simulink model "MPC_circle_tracking"  (R2023a)
settings: Solver=VariableStepAuto  StartTime=0.0  StopTime=40  FixedStep=0.001  RelTol=1e-3
libraries: slpidlib x2, Solver_SF x1
settings Model: Creator=ASUS  LastModifiedBy=69546
settings SolverCC: AlgebraicLoopSolver=TrustRegion
settings DebuggingCC: UnconnectedInputMsg=warning  UnconnectedOutputMsg=warning  UnconnectedLineMsg=warning
settings ModelReferenceCC: EnableRefExpFcnMdlSchedulingChecks=on
settings SFSimCC: CustomCodeUndefinedFunction=UseInterfaceOnly

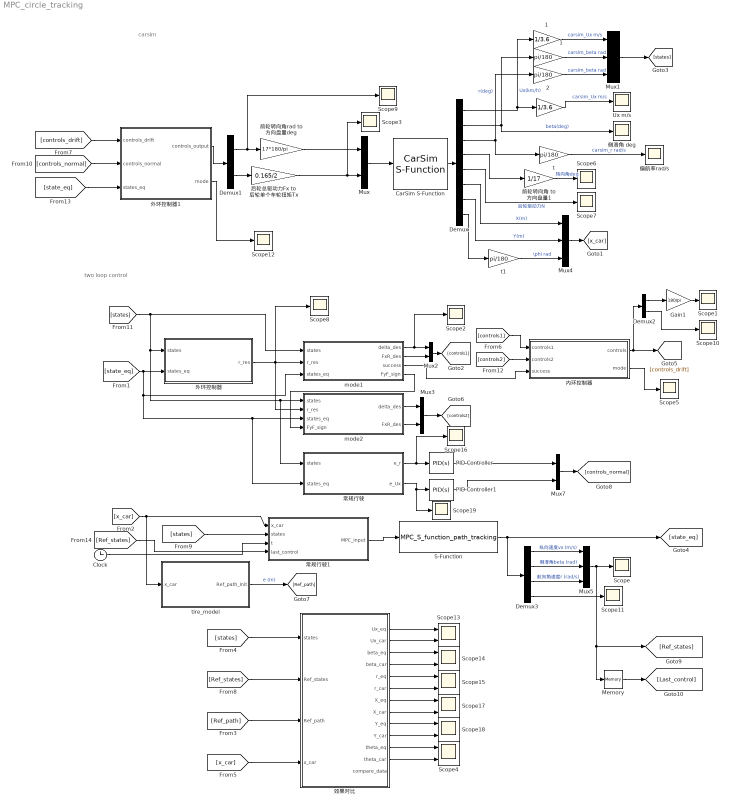
== system MPC_circle_tracking ==
  note: carsim
  note: two loop control
  " " : Gain  Gain=1/3.6
  " 1" : Gain  Gain=1/3.6
  " 1" : Gain  Gain=pi/180
  " 2" : Gain  Gain=pi/180
  " t" : Gain  Gain=pi/180
  " t1" : Gain  Gain=pi/180
  CarSim S-Function : Solver_SF/CarSim S-Function  Priority=1  SIMFILE=simfile.sim  Run_RTs=off  vs_state_ind=Run  StopMode_ind=Vehicle Model
  Clock : Clock
  Demux : Demux  Outputs=8
  Demux1 : Demux  Outputs=[1 1]
  Demux2 : Demux  Outputs=2
  Demux3 : Demux
  Gain1 : Gain  Gain=180/pi
  Memory : Memory
  Mux{,2..3,7} (4 alike) : Mux  Inputs=2
  Mux1 : Mux  Inputs=3
  Mux4 : Mux  Inputs=3
  Mux5 : Mux  Inputs=3
  PID Controller : slpidlib/PID Controller  Controller=PID  Form=Parallel  TimeDomain=Continuous-time  UseExternalTs=off  SampleTime=-1  IntegratorMethod=Forward Euler  FilterMethod=Forward Euler  ControllerParametersSource=internal  P=3  I=1  UseKiTs=off  D=0  N=100  UseFilter=on  TunerSelectOption=Transfer Function Based (PID Tuner App)  InitialConditionSource=internal  InitialConditionForIntegrator=0  InitialConditionForFilter=0  DifferentiatorICPrevScaledInput=0  ExternalReset=none  TrackingMode=off  Kt=1  LimitOutput=on  SatLimitsSource=internal  UpperSaturationLimit=30*pi/180  LowerSaturationLimit=-30*pi/180  LinearizeAsGain=off  AntiWindupMode=none  Kb=1  LimitIntegrator=off  UpperIntegratorSaturationLimit=inf  LowerIntegratorSaturationLimit=-inf  POutMin=[]  POutMax=[]  IOutMin=[]  IOutMax=[]  DOutMin=[]  DOutMax=[]  NOutMin=[]  NOutMax=[]  SumOutMin=[]  SumOutMax=[]  SaturationOutMin=[]  SaturationOutMax=[]  PParamMin=[]  PParamMax=[]  IParamMin=[]  IParamMax=[]  DParamMin=[]  DParamMax=[]  NParamMin=[]  NParamMax=[]  KbParamMin=[]  KbParamMax=[]  KtParamMin=[]  KtParamMax=[]  KbOutMin=[]  KbOutMax=[]  KtOutMin=[]  KtOutMax=[]  IntegratorOutMin=[]  IntegratorOutMax=[]  FilterOutMin=[]  FilterOutMax=[]  SumI1OutMin=[]  SumI1OutMax=[]  SumI2OutMin=[]  SumI2OutMax=[]  SumI3OutMin=[]  SumI3OutMax=[]  SumI4OutMin=[]  SumI4OutMax=[]  SumDOutMin=[]  SumDOutMax=[]  DifferentiatorOutMin=[]  DifferentiatorOutMax=[]  FilterDiffOutCoefMin=[]  FilterDiffOutCoefMax=[]  ReciprocalOutMin=[]  ReciprocalOutMax=[]  SumDenOutMin=[]  SumDenOutMax=[]  SumNumOutMin=[]  SumNumOutMax=[]  DivideOutMin=[]  DivideOutMax=[]  UdiffTsProdOutMin=[]  UdiffTsProdOutMax=[]  NTsProdOutMin=[]  NTsProdOutMax=[]  UintegralTsProdOutMin=[]  UintegralTsProdOutMax=[]  UngainTsProdOutMin=[]  UngainTsProdOutMax=[]  ClampingZeroOutDataTypeStr=Inherit: Inherit via back propagation  ClampingZeroOutMin=[]  ClampingZeroOutMax=[]  FilterDenConstantOutDataTypeStr=Inherit: Inherit via back propagation  FilterDenConstantOutMin=[]  FilterDenConstantOutMax=[]  PCopyOutDataTypeStr=Inherit: Inherit via back propagation  PCopyOutMin=[]  PCopyOutMax=[]  NCopyOutDataTypeStr=Inherit: Inherit via back propagation  NCopyOutMin=[]  NCopyOutMax=[]  IntegratorContinuousStateAttributes=''  IntegratorStateMustResolveToSignalObject=off  IntegratorRTWStateStorageClass=Auto  FilterContinuousStateAttributes=''  FilterStateMustResolveToSignalObject=off  FilterRTWStateStorageClass=Auto  ParallelPVariant=InternalParameters  IdealPVariant=Disabled  IVariant=InternalParameters  DVariant=InternalParameters  IntegratorVariant=Continuous  SatVariant=Enabled  AWVariant=Passthrough  PCopyVariant=Disabled  TRVariant=Disabled  FdbkBlocksVariant=Forward  IdealPFdbkVariant=Disabled  SatFdbkVariant=Disabled  DerivativeFilterVariant=ContFilter  NVariant=InternalParameters  NCopyVariant=Disabled  FilterICVariant=InternalICsFilter  IntegratorICVariant=InternalICs  ExternalResetVariant=Disabled  TRSumVariant=Passthrough  SumFdbkVariant=Disabled  SumVariant=Sum_PID  TsampFilterVariant=InternalTs  TsampNgainVariant=Passthrough  TsampIntegralVariant=Disabled_SignalSpec  ExternalSaturationOutDataTypeStr=Inherit: Same as second input
  PID Controller1 : slpidlib/PID Controller  Controller=PID  Form=Parallel  TimeDomain=Continuous-time  UseExternalTs=off  SampleTime=-1  IntegratorMethod=Forward Euler  FilterMethod=Forward Euler  ControllerParametersSource=internal  P=1000  I=50  UseKiTs=off  D=0  N=100  UseFilter=on  TunerSelectOption=Transfer Function Based (PID Tuner App)  InitialConditionSource=internal  InitialConditionForIntegrator=0  InitialConditionForFilter=0  DifferentiatorICPrevScaledInput=0  ExternalReset=none  TrackingMode=off  Kt=1  LimitOutput=on  SatLimitsSource=internal  UpperSaturationLimit=4000  LowerSaturationLimit=-4000  LinearizeAsGain=on  AntiWindupMode=none  Kb=1  LimitIntegrator=off  UpperIntegratorSaturationLimit=inf  LowerIntegratorSaturationLimit=-inf  POutMin=[]  POutMax=[]  IOutMin=[]  IOutMax=[]  DOutMin=[]  DOutMax=[]  NOutMin=[]  NOutMax=[]  SumOutMin=[]  SumOutMax=[]  SaturationOutMin=[]  SaturationOutMax=[]  PParamMin=[]  PParamMax=[]  IParamMin=[]  IParamMax=[]  DParamMin=[]  DParamMax=[]  NParamMin=[]  NParamMax=[]  KbParamMin=[]  KbParamMax=[]  KtParamMin=[]  KtParamMax=[]  KbOutMin=[]  KbOutMax=[]  KtOutMin=[]  KtOutMax=[]  IntegratorOutMin=[]  IntegratorOutMax=[]  FilterOutMin=[]  FilterOutMax=[]  SumI1OutMin=[]  SumI1OutMax=[]  SumI2OutMin=[]  SumI2OutMax=[]  SumI3OutMin=[]  SumI3OutMax=[]  SumI4OutMin=[]  SumI4OutMax=[]  SumDOutMin=[]  SumDOutMax=[]  DifferentiatorOutMin=[]  DifferentiatorOutMax=[]  FilterDiffOutCoefMin=[]  FilterDiffOutCoefMax=[]  ReciprocalOutMin=[]  ReciprocalOutMax=[]  SumDenOutMin=[]  SumDenOutMax=[]  SumNumOutMin=[]  SumNumOutMax=[]  DivideOutMin=[]  DivideOutMax=[]  UdiffTsProdOutMin=[]  UdiffTsProdOutMax=[]  NTsProdOutMin=[]  NTsProdOutMax=[]  UintegralTsProdOutMin=[]  UintegralTsProdOutMax=[]  UngainTsProdOutMin=[]  UngainTsProdOutMax=[]  ClampingZeroOutDataTypeStr=Inherit: Inherit via back propagation  ClampingZeroOutMin=[]  ClampingZeroOutMax=[]  FilterDenConstantOutDataTypeStr=Inherit: Inherit via back propagation  FilterDenConstantOutMin=[]  FilterDenConstantOutMax=[]  PCopyOutDataTypeStr=Inherit: Inherit via back propagation  PCopyOutMin=[]  PCopyOutMax=[]  NCopyOutDataTypeStr=Inherit: Inherit via back propagation  NCopyOutMin=[]  NCopyOutMax=[]  IntegratorContinuousStateAttributes=''  IntegratorStateMustResolveToSignalObject=off  IntegratorRTWStateStorageClass=Auto  FilterContinuousStateAttributes=''  FilterStateMustResolveToSignalObject=off  FilterRTWStateStorageClass=Auto  ParallelPVariant=InternalParameters  IdealPVariant=Disabled  IVariant=InternalParameters  DVariant=InternalParameters  IntegratorVariant=Continuous  SatVariant=Enabled  AWVariant=Passthrough  PCopyVariant=Disabled  TRVariant=Disabled  FdbkBlocksVariant=Forward  IdealPFdbkVariant=Disabled  SatFdbkVariant=Disabled  DerivativeFilterVariant=ContFilter  NVariant=InternalParameters  NCopyVariant=Disabled  FilterICVariant=InternalICsFilter  IntegratorICVariant=InternalICs  ExternalResetVariant=Disabled  TRSumVariant=Passthrough  SumFdbkVariant=Disabled  SumVariant=Sum_PID  TsampFilterVariant=InternalTs  TsampNgainVariant=Passthrough  TsampIntegralVariant=Disabled_SignalSpec  ExternalSaturationOutDataTypeStr=Inherit: Same as second input
  S-Function : S-Function  FunctionName=MPC_S_function_path_tracking  SFunctionDeploymentMode=off  EnableBusSupport=off
  Scope{,1..3,5..12,16,19} (14 alike) : Scope
  Scope{4,13..15,17..18} (6 alike) : Scope  NumInputPorts=2
  Ux m/s : Scope
  mode1 : MATLAB Function  TreatAsAtomicUnit=on
  mode2 : MATLAB Function  TreatAsAtomicUnit=on
  tire_model : MATLAB Function  TreatAsAtomicUnit=on
  侧滑角 deg : Scope
  偏航率rad/s : Scope
  内环控制器 : MATLAB Function  TreatAsAtomicUnit=on
  前轮转向角 to 方向盘量1 : Gain  Gain=1/17
  前轮转向角rad to 方向盘量deg : Gain  Gain=17*180/pi
  后轮总驱动力Fx to 后轮单个车轮扭矩Tx : Gain  Gain=0.165/2
  外环控制器 : MATLAB Function  TreatAsAtomicUnit=on
  外环控制器1 : MATLAB Function  TreatAsAtomicUnit=on
  常规行驶 : MATLAB Function  TreatAsAtomicUnit=on
  常规行驶1 : MATLAB Function  TreatAsAtomicUnit=on
  效果对比 : MATLAB Function  TreatAsAtomicUnit=on
  wires:
  内环控制器/1(controls) -> [controls_drift], Demux2/1
  mode1/1(delta_des) -> Scope2/1, Mux2/1
  Gain1/1 -> Scope1/1
  Demux2/2 -> Scope10/1
  Mux2/1 -> [controls1]
  Demux2/1 -> Gain1/1
  [controls2] -> 内环控制器/2(controls2)
  [states] -> 常规行驶/1(states), mode2/1(states), 外环控制器/1(states), mode1/1(states)
  mode2/1(delta_des) -> Mux3/1
  mode1/2(FxR_des) -> Mux2/2
  Mux3/1 -> [controls2]
  mode2/2(FxR_des) -> Mux3/2
  内环控制器/2(mode) -> Scope5/1
  mode1/3(success) -> 内环控制器/3(success)
  [controls1] -> 内环控制器/1(controls1)
  外环控制器/1(r_res) -> mode2/2(r_res), mode1/2(r_res), Scope8/1
  " t"/1 -> 偏航率rad/s/1  "carsim_r rad/s"
  " "/1 -> Ux m/s/1  "carsim_Ux m/s"
  " 1"/1 -> Mux1/2  "carsim_beta rad"
  " 2"/1 -> Mux1/3  "carsim_beta rad"
  Demux1/2 -> 后轮总驱动力Fx to 后轮单个车轮扭矩Tx/1
  Demux/1 -> " 1"/1, " "/1  "Ux(km/h)"
  Demux/5 -> Scope7/1  "后轮驱动力N"
  Demux/4 -> 前轮转向角 to 方向盘量1/1
  Mux/1 -> CarSim S-Function/1
  Mux1/1 -> [states]
  CarSim S-Function/1 -> Demux/1
  " 1"/1 -> Mux1/1  "carsim_Ux m/s"
  前轮转向角 to 方向盘量1/1 -> Scope6/1  "转向角deg"
  Demux/3 -> " 2"/1, " t"/1  "r(deg)"
  Demux/2 -> " 1"/1, 侧滑角 deg/1  "beta(deg)"
  Demux1/1 -> Scope9/1, 前轮转向角rad to 方向盘量deg/1
  mode1/4(FyF_sign) -> mode2/4(FyF_sign)
  Demux/8 -> " t1"/1
  " t1"/1 -> Mux4/3  "\\phi rad"
  Mux4/1 -> [x_car]
  [state_eq] -> 常规行驶/2(states_eq), mode2/3(states_eq), mode1/3(states_eq), 外环控制器/2(states_eq)
  S-Function/1 -> Demux3/1, [state_eq]
  Demux/6 -> Mux4/1  "X(m)"
  Demux/7 -> Mux4/2  "Y(m)"
  Demux3/1 -> Mux5/1  "纵向速度vx (m/s)"
  Demux3/2 -> Mux5/2  "侧滑角beta (rad)"
  Demux3/3 -> Mux5/3  "航向角速度r (rad/s)"
  Mux5/1 -> Memory/1, [Ref_states], Scope/1
  常规行驶/1(e_r) -> Scope16/1, PID Controller/1
  常规行驶/2(e_Ux) -> Scope19/1, PID Controller1/1
  Mux7/1 -> [controls_normal]
  常规行驶1/1(MPC_input) -> S-Function/1
  tire_model/1(Ref_path_Init) -> [Ref_path]  "e (m)"
  [x_car] -> tire_model/1(x_car), 常规行驶1/1(x_car)
  效果对比/4(beta_car) -> Scope14/2
  效果对比/6(r_car) -> Scope15/2
  效果对比/8(X_car) -> Scope17/2
  效果对比/7(X_eq) -> Scope17/1
  效果对比/11(theta_eq) -> Scope4/1
  效果对比/12(theta_car) -> Scope4/2
  [x_car] -> 效果对比/4(x_car)
  效果对比/10(Y_car) -> Scope18/2
  效果对比/3(beta_eq) -> Scope14/1
  效果对比/9(Y_eq) -> Scope18/1
  [states] -> 效果对比/1(states)
  效果对比/5(r_eq) -> Scope15/1
  效果对比/2(Ux_car) -> Scope13/2
  [Ref_path] -> 效果对比/3(Ref_path)
  效果对比/1(Ux_eq) -> Scope13/1
  Demux3/4 -> Scope11/1
  PID Controller1/1 -> Mux7/2
  Clock/1 -> 常规行驶1/3(t)
  后轮总驱动力Fx to 后轮单个车轮扭矩Tx/1 -> Scope3/1, Mux/2
  前轮转向角rad to 方向盘量deg/1 -> Mux/1
  [Ref_states] -> 效果对比/2(Ref_states)
  [states] -> 常规行驶1/2(states)
  [controls_drift] -> 外环控制器1/1(controls_drift)
  外环控制器1/1(controls_output) -> Demux1/1
  [controls_normal] -> 外环控制器1/2(controls_normal)
  [state_eq] -> 外环控制器1/3(states_eq)
  外环控制器1/2(mode) -> Scope12/1
  PID Controller/1 -> Mux7/1
  [Ref_states] -> 常规行驶1/4(last_control)
  Memory/1 -> [Last_control]

== matlab function MPC_circle_tracking/效果对比 ==
  data: Ux_eq output; states input; Ref_states input; Ref_path input; x_car input; Ux_car output; beta_eq output; beta_car output; r_eq output; r_car output; X_eq output; X_car output; Y_eq output; Y_car output; theta_eq output; theta_car output; compare_data output
 function [Ux_eq,Ux_car,beta_eq,beta_car,r_eq,r_car,X_eq,X_car,Y_eq,Y_car,theta_eq,theta_car,compare_data] = output_compare(states,Ref_states,Ref_path,x_car)
        %期望值
        
        X_eq=Ref_path(1);
        Y_eq=Ref_path(2);
        theta_eq=Ref_path(3);
        Ux_eq=Ref_path(4);
        beta_eq=atan2(Ref_path(5),Ux_eq);
        r_eq=Ref_path(6);
        % Ux_eq=Ref_states(1);
        % beta_eq=Ref_states(2);
        % r_eq=Ref_states(3);
        V_eq=Ux_eq/( cos(beta_eq)+eps );
        %实际值
        Ux_car=states(1);
        beta_car=states(2);
        r_car=states(3);
        
        X_car=x_car(1);
        Y_car=x_car(2);
        theta_car=x_car(3);

        V_car=Ux_car/( cos(beta_car)+eps );
        compare_data=[Ux_eq,Ux_car,beta_eq,beta_car,r_eq,r_car,X_eq,X_car,Y_eq,Y_car,theta_eq,theta_car] ;
        
end

== matlab function MPC_circle_tracking/外环控制器1 ==
  data: controls_output output; controls_drift input; controls_normal input; states_eq input; mode output
function [controls_output,mode] = outloop_control(controls_drift,controls_normal,states_eq)
        %车辆参数及控制器相关参数都在car_parameters文件中配置
        beta_eq=states_eq(2)   ;
        %常规控制器
        if abs(beta_eq)<0.2
            controls_output=controls_normal;
            mode=0;
         %漂移控制器
        else
            controls_output=controls_drift;
            mode=1;
        end

        
end

== matlab function MPC_circle_tracking/常规行驶 ==
  data: e_r output; states input; e_Ux output; states_eq input

function [e_r,e_Ux] = normal(states,states_eq)


    Ux_eq=states_eq(1)    ;
    beta_eq=states_eq(2)    ;
    r_eq=states_eq(3) ;

    Ux = states(1);
    beta=states(2)    ;
    r = states(3);

    e_Ux = -(Ux-Ux_eq);
    e_r = -(r-r_eq)-1*(beta-beta_eq);


end

== matlab function MPC_circle_tracking/tire_model ==
  data: Ref_path_Init output; x_car input
function Ref_path_Init  = tire_model(x_car)
    Ref_path_Init=[0;0;0;0;0;0] ;
    currentPosition=[x_car(1),x_car(2)];
    nearestPoint = findNearestPoint(currentPosition,x_car(3),0);
    %初始最近跟踪匹配点
    X_r=nearestPoint(1);
    Y_r=nearestPoint(2);
    theta_r=nearestPoint(3);  
    Ux_r=nearestPoint(4);
    Uy_r=nearestPoint(5);
    r_r=nearestPoint(6);  
    %最近跟踪点的参考车辆状态
    Ref_path_Init(1)=X_r;
    Ref_path_Init(2)=Y_r;
    Ref_path_Init(3)=theta_r;  
    Ref_path_Init(4)=Ux_r;
    Ref_path_Init(5)=Uy_r;
    Ref_path_Init(6)=r_r;  

             
end

== matlab function MPC_circle_tracking/内环控制器 ==
  data: controls output; controls1 input; controls2 input; success input; mode output
function [controls, mode] = innerloop_control(controls1,controls2,success)
    % Mode 2 - Drive force mode
    if success
        controls=controls1;
        mode = 1;
    else
        controls=controls2;
        mode = 2;
    end
    
end

== matlab function MPC_circle_tracking/mode1 ==
  data: delta_des output; states input; FxR_des output; success output; r_res input; states_eq input; FyF_sign output
function [delta_des,FxR_des,success,FyF_sign] = mode1(states,r_res,states_eq)
    %车辆参数及控制器相关参数都在car_parameters文件中配置
    pars = car_parameters();
    % Extract parameters and control constants
    a = pars.a;
    b = pars.b;
    m = pars.m;
    mu = pars.mu;
    B=pars.B;      % N / rad
    C=pars.C;      % N / rad
    Iz = pars.Iz;
    Fz = pars.Fz;
    FzF = pars.FzF;
    FzR = pars.FzR;

    K_beta = pars.K_beta;
    K_r = pars.K_r;
    K_Ux = pars.K_Ux;
    
    Ux_eq=states_eq(1)    ;
    beta_eq=states_eq(2)   ;
    r_eq=states_eq(3) ;
    FxR_eq=states_eq(4); 
    

    FxR_max = pars.FxR_max;
    delta_max = pars.delta_max;
    L = pars.L; % m
    CaF = pars.CaF;      % N / rad
    CaR = pars.CaR;      % N / rad
    % Extract states and errors

    Ux = states(1);
    beta = states(2);
    r = states(3);
 
    e_Ux = Ux-Ux_eq;
    e_beta= beta-beta_eq;
    e_r = r-r_res;
    

    % Compute constants
    k1 = a/Iz - K_beta / (m * Ux);
    k2 = b/Iz + K_beta / (m * Ux);

    % Compute desired rear drive force and resulting lateral force
    FxR_des = FxR_eq - m * K_Ux * e_Ux;
    FxR_des = min(FxR_des, FxR_max);
    FxR_des = max(FxR_des, 0);
    % Compute rear lateral force based on current state
    % FyR_des = a*m/L*r*Ux;   % Page 42 of Thesis - is this valid for normal use? 
    aR=atan(tan(beta)-(b*r)/Ux);
    %计算后轮极限侧偏角(mu*FzR)^2-FxR_des^2   
    acr=tan(asin(sqrt((mu*FzR)^2-FxR_des^2)/(mu*FzR))/C)/B;
    %判断后轮是否饱和，若饱和则后轮侧向力受纵向力影响

    if abs(aR)<abs(acr)
        FyR_des=-1*mu*FzR*sin(C*atan(B*aR))*2/3;
    else
        FyR_des=-1*sqrt((mu*FzR)^2-FxR_des^2)*sign(aR)*2/3;
    end 

    % Compute desired front lateral force
    FyF_des = 1/k1 * ( k2 * FyR_des - K_beta^2 * e_beta - K_beta * r_eq -(K_beta + K_r) * e_r );

    % Compute desired steering angle if this is possible
    if  abs(FyF_des)< mu*FzF
        % Compute desired steering angle
        aF=tan(asin( FyF_des/(-mu*FzF))/C)/B;
        delta_des=(atan(beta+(a*r)/Ux)-aF);
        delta_des = min(delta_des, delta_max);
        delta_des = max(delta_des, -delta_max);
        success = true;
        
    else
        delta_des = NaN;
        success = false;
    end
    FyF_sign=sign(FyF_des);
end

== matlab function MPC_circle_tracking/常规行驶1 ==
  data: MPC_input output; x_car input; states input; t input; last_control input

function MPC_input = mux(x_car,states,t,last_control)
   MPC_input=zeros(10,1);
   MPC_input(1)=x_car(1);
   MPC_input(2)=x_car(2);

   MPC_input(3)=x_car(3);
   MPC_input(4)=states(1);
   MPC_input(5)=states(2);
   MPC_input(6)=states(3);
   MPC_input(7)=t;

   MPC_input(8)=last_control(1);
   MPC_input(9)=last_control(2);
   MPC_input(10)=last_control(3);

  
end

== matlab function MPC_circle_tracking/外环控制器 ==
  data: r_res output; states input; states_eq input
function r_res = outloop_control(states,states_eq)
        %车辆参数及控制器相关参数都在car_parameters文件中配置
        pars = car_parameters(); 
        K_beta=pars.K_beta;
        
        Ux_eq=states_eq(1)    ;
        beta_eq=states_eq(2)   ;
        r_eq=states_eq(3) ;
        FxR_eq=states_eq(4); 
        
        beta=states(2);
         %对侧滑角进行前馈和反馈控制，输出期望航向角速度给内环控制器
        r_res=r_eq+K_beta*(beta-beta_eq);
        
end

== matlab function MPC_circle_tracking/mode2 ==
  data: delta_des output; states input; FxR_des output; r_res input; states_eq input; FyF_sign input

function [delta_des,FxR_des] = mode2(states,r_res,states_eq,FyF_sign)
    % Extract parameters and control constants
    %车辆参数及控制器相关参数都在car_parameters文件中配置
    pars = car_parameters();
    a = pars.a;
    b = pars.b;
    m = pars.m;
    mu = pars.mu;
    B=pars.B;      % N / rad
    C=pars.C;      % N / rad
    Iz = pars.Iz;
    Fz = pars.Fz;
    FzF = pars.FzF;
    FzR = pars.FzR;

    K_beta = pars.K_beta;
    K_r = pars.K_r;
    K_Ux = pars.K_Ux;
    
    Ux_eq=states_eq(1)    ;
    beta_eq=states_eq(2)   ;
    r_eq=states_eq(3) ;
    FxR_eq=states_eq(4);      
    %改变稳态值


    FxR_max = pars.FxR_max;
    delta_max = pars.delta_max;
    L = pars.L; % m
    CaF = pars.CaF;      % N / rad
    CaR = pars.CaR;      % N / rad
    % Extract states and errors
    
    Ux = states(1);
    beta = states(2);
    r = states(3);

    e_Ux = Ux-Ux_eq;
    e_beta= beta-beta_eq;
    e_r = r-r_res;

    % Compute constants
    
    k1 = a/Iz - K_beta / (m * Ux);
    k2 = b/Iz + K_beta / (m * Ux);
    
    % Compute desired front lateral force - saturated
    FyF_des = FyF_sign*mu * FzF;
    
    % Compute desired rear lateral force
    FyR_des = 1/k2 * (k1 * mu * FzF + K_beta^2 * e_beta + K_beta * r_eq + (K_beta + K_r) * e_r );
    FyR_des = min(FyR_des, mu*FzR);
    FyR_des = max(FyR_des, -mu*FzR);
    
    % Compute desired rear longitudinal force
    FxR_des = sqrt((mu*FzR)^2 - (FyR_des)^2);
    FxR_des = min(FxR_des, FxR_max);
    FxR_des = max(FxR_des, 0);
        
    if ~isreal(FxR_des)
        error('Mode 2 Error: FyR_des is larger than mu*FzR')
    end
    
    % Compute desired steering angle
    aF=tan(asin(FyF_des/(-mu*FzF))/C)/B;
    delta_des=(atan(beta+(a*r)/Ux)-aF);
    delta_des = min(delta_des, delta_max);
    delta_des = max(delta_des, -delta_max);
end
